simulink model "sim1"  (R2015a)
settings: Solver=ode45  StartTime=0.0  StopTime=10.0  RelTol=1e-3
settings Model: Creator=Asus  LastModifiedBy=Asus

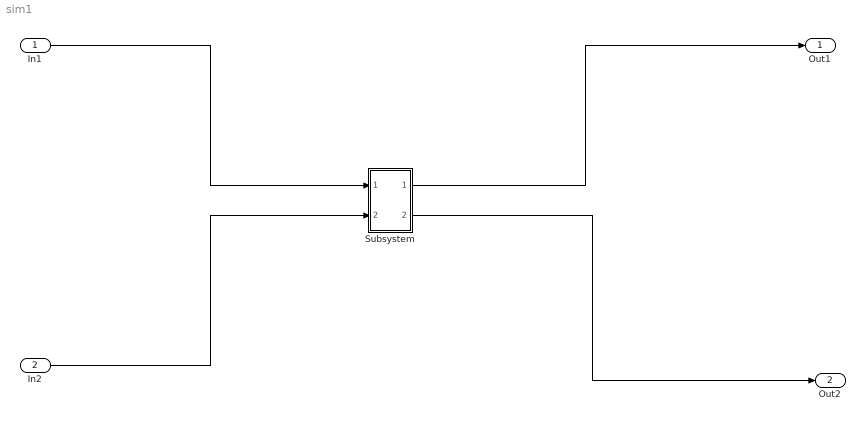
== system sim1 ==
  In1 : Inport
  In2 : Inport  Port=2
  Subsystem : Subsystem
  Out1 : Outport
  Out2 : Outport  Port=2
  wires:
  In1/1 -> Subsystem/1(In1)
  In2/1 -> Subsystem/2(In2)
  Subsystem/1(Out1) -> Out1/1
  Subsystem/2(Out2) -> Out2/1

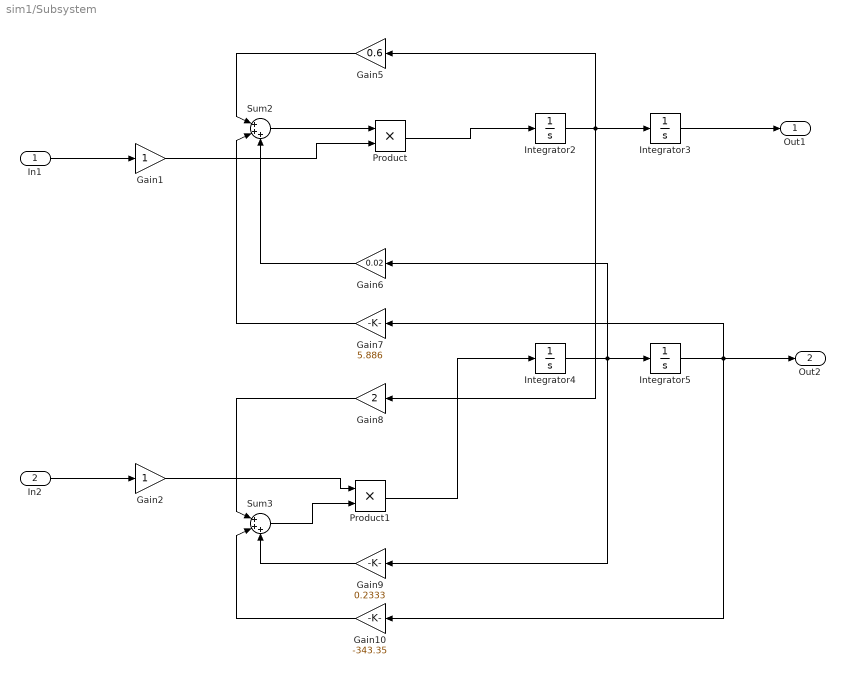
== system sim1/Subsystem ==
  In1 : Inport
  In2 : Inport  Port=2
  Gain1 : Gain
  Gain10 : Gain  Gain=-343.35
  Gain2 : Gain
  Gain5 : Gain  Gain=0.6
  Gain6 : Gain  Gain=0.02
  Gain7 : Gain  Gain=5.886
  Gain8 : Gain  Gain=2
  Gain9 : Gain  Gain=0.2333
  Integrator{2..5} (4 alike) : Integrator
  Product : Product
  Product1 : Product
  Sum2 : Sum  Inputs=|+++
  Sum3 : Sum  Inputs=|+++
  Out1 : Outport
  Out2 : Outport  Port=2
  wires:
  Integrator2/1 -> Gain8/1, Gain5/1, Integrator3/1
  In1/1 -> Gain1/1
  Gain1/1 -> Product/2
  Integrator3/1 -> Out1/1
  Gain9/1 -> Sum3/3
  Gain10/1 -> Sum3/2
  Gain8/1 -> Sum3/1
  Sum2/1 -> Product/1
  Product/1 -> Integrator2/1
  Gain7/1 -> Sum2/2
  Gain6/1 -> Sum2/3
  In2/1 -> Gain2/1
  Integrator5/1 -> Out2/1, Gain10/1, Gain7/1
  Sum3/1 -> Product1/2
  Gain2/1 -> Product1/1
  Product1/1 -> Integrator4/1
  Integrator4/1 -> Gain9/1, Gain6/1, Integrator5/1
  Gain5/1 -> Sum2/1
